simulink model "NetraScan_Simulink"  (R2026a)
settings: Solver=VariableStepAuto  StopTime=1000
libraries: simulink x1, visionsources x1
settings Model: Creator=riteshtiwari06  LastModifiedBy=riteshtiwari06
settings DebuggingCC: UnitsInconsistencyMsg=none

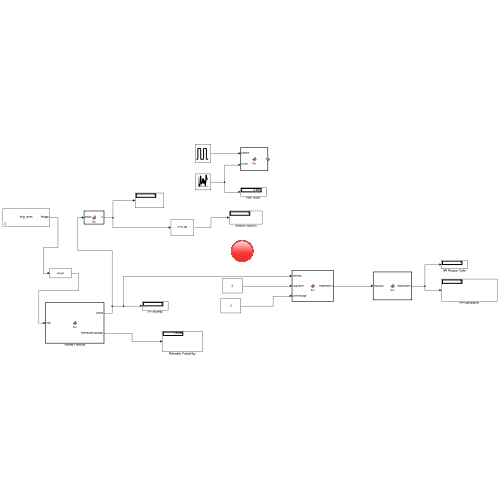
[thumbnail: Simulink's stored preview of the top-level diagram]
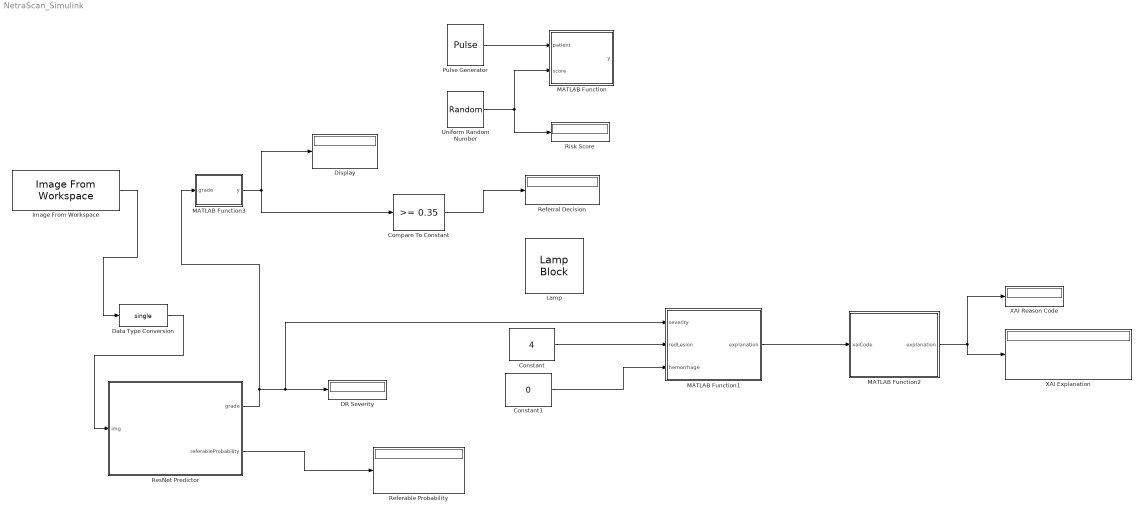
== system NetraScan_Simulink ==
  Compare To Constant : simulink/Logic and Bit Operations/Compare To Constant  relop=>=  const=0.35  OutDataTypeStr=boolean
  Constant : Constant  Value=4
  Constant1 : Constant  Value=0
  DR Severity : Display
  Data Type Conversion : DataTypeConversion  OutDataTypeStr=single  SaturateOnIntegerOverflow=off  RndMeth=Floor
  Display : Display
  Image From Workspace : visionsources/Image From Workspace  Tag=vipblks_nd  ImageValue=img_norm  Ts=1  imagePorts=One multidimensional signal  OutPortLabels=R|G|B  ImageDataType=Inherit from 'Value'  Signed=on  WordLength=16  sdImageDataType=sfix(16)  FractionLengthMode=User-defined  FractionLength=15
  Lamp : LampBlock  LabelPosition=Hide  DefaultColor=[192.0, 192.0, 192.0]
  MATLAB Function : MATLAB Function  TreatAsAtomicUnit=on
  MATLAB Function1 : MATLAB Function  TreatAsAtomicUnit=on
  MATLAB Function2 : MATLAB Function  TreatAsAtomicUnit=on
  MATLAB Function3 : MATLAB Function  TreatAsAtomicUnit=on
  Pulse Generator : DiscretePulseGenerator  PulseType=Time based  Period=106
  Referable Probability : Display
  Referral Decision : Display
  ResNet Predictor : MATLAB Function  TreatAsAtomicUnit=on
  Risk Score : Display
  Uniform Random Number : UniformRandomNumber  Minimum=0  Maximum=10  Seed=00001  SampleTime=1
  XAI Explanation : Display
  XAI Reason Code : Display
  wires:
  Pulse Generator/1 -> MATLAB Function/1(patient)
  Uniform Random Number/1 -> Risk Score/1, MATLAB Function/2(score)
  Compare To Constant/1 -> Referral Decision/1
  Constant1/1 -> MATLAB Function1/3(hemorrhage)
  MATLAB Function1/1(explanation) -> MATLAB Function2/1(xaiCode)
  MATLAB Function2/1(explanation) -> XAI Reason Code/1, XAI Explanation/1
  Image From Workspace/1 -> Data Type Conversion/1
  MATLAB Function3/1(y) -> Compare To Constant/1, Display/1
  ResNet Predictor/1(grade) -> MATLAB Function3/1(grade), MATLAB Function1/1(severity), DR Severity/1
  Data Type Conversion/1 -> ResNet Predictor/1(img)
  Constant/1 -> MATLAB Function1/2(redLesion)
  ResNet Predictor/2(referableProbability) -> Referable Probability/1

== matlab function NetraScan_Simulink/MATLAB Function1 ==
  data: severity input; explanation output; redLesion input; hemorrhage input
function explanation = fcn(severity, redLesion, hemorrhage)
%#codegen

if severity >= 2 && redLesion == 1
    explanation = 1;      % Referral + red lesions
elseif severity >= 2 && hemorrhage == 1
    explanation = 2;      % Referral + hemorrhage
elseif severity >= 2
    explanation = 3;      % Referral due to severity
elseif severity == 1
    explanation = 4;      % Mild DR
else
    explanation = 0;      % No significant finding
end

== matlab function NetraScan_Simulink/MATLAB Function ==
  data: y output; patient input; score input
function y = fcn(patient, score)

%#codegen

% ResNet predicted grade is already 0-4
y = floor(score);

end

== matlab function NetraScan_Simulink/MATLAB Function2 ==
  data: xaiCode input; explanation output
function explanation = fcn(xaiCode)
%#codegen

if xaiCode == 0
    explanation = 0;   % No significant finding
elseif xaiCode == 1
    explanation = 1;   % Red lesion contributed
elseif xaiCode == 2
    explanation = 2;   % Hemorrhage contributed
elseif xaiCode == 3
    explanation = 3;   % Severity caused referral
else
    explanation = 4;   % Mild DR
end

== matlab function NetraScan_Simulink/MATLAB Function3 ==
  data: grade input; y output
function y = fcn(grade)
%#codegen

if grade >= 2
    y = true;
else
    y = false;
end

== matlab function NetraScan_Simulink/ResNet Predictor ==
  data: img input single size=[224 224 3]; grade output double size=[1 1]; referableProbability output
function [grade, referableProbability] = fcn(img)
%#codegen

coder.extrinsic('NetraScan_SimulinkInference');

grade = double(0);
referableProbability = double(0);

[grade, ~, referableProbability] = ...
    NetraScan_SimulinkInference(img);

end
